simulink library "tqd"  (R2021b)
settings: Solver=VariableStepAuto  StartTime=0.0  StopTime=10.0  RelTol=1e-3
undefined symbols (not defined in the file or in its folder): ATQD_APSDecReq_X_kph, ATQD_APSDecReq_Y_mps2, ATQD_APSDecReqCMD_X_kph, ATQD_APSDecReqTs_X_pct, ATQD_APSDecTimeGain_X_Deg, ATQD_APSDecTimeGain_Y_s, ATQD_APSReqLowSpd_X_Deg, ATQD_AutoHoldReleaseBPS_X_Deg, ATQD_AWDLoadTrqnsGain_X_kg, ATQD_AWDLoadTrqnsGain_Y_pct, ATQD_BOSEnBPSPosn_X_kph, ATQD_BOSMap_X_rpm, ATQD_BOSMap_Y_pct, ATQD_CreepBaseTqD_X_kph, ATQD_CreepBaseTqD_Y_Deg, ATQD_CreepBaseTqR_X_kph, ATQD_CreepBaseTqR_Y_Deg, ATQD_CreepBPSDisPosn_X_Deg, ATQD_CreepBPSDisPosnR_X_Deg, ATQD_CreepBPSEnPosn_X_Deg, ATQD_CreepBPSEnPosnR_X_Deg, ATQD_CreepDeltaTq_X_kph, ATQD_CreepIterm_X_kph, ATQD_CreepIterm_Y_kph, ATQD_CreepItermMaxLimit_X_pct, ATQD_CreepPreloadTime_X_kph, ATQD_CreepPreloadTq_X_kph, ATQD_CreepPreloadTq_Y_s, ATQD_CreepProtTq_X_Deg, ATQD_CreepPterm_X_kph, ATQD_CreepPterm_Y_kph, ATQD_ECOTqMapD_X_rpm, ATQD_ECOTqMapD_Y_pct, ATQD_EOPDTqMapDCon_X_rpm, ATQD_EOPDTqMapDCon_Y_Deg, ATQD_EstInitVehWeight_X_c, ATQD_LHMRollGenMapD_X_rpm, ATQD_LHMRollGenMapD_Y_rpm, ATQD_LHMTqMapD_X_rpm, ATQD_LHMTqMapD_Y_pct, ATQD_NL1TqMapD_X_rpm, ATQD_NL1TqMapD_Y_pct, ATQD_NOPDTqMapDCon_X_rpm, ATQD_NOPDTqMapDCon_Y_Deg, ATQD_NRMRrEDUSpRat_X_rpm, ATQD_NRMRrEDUSpRat_Y_Nm, ATQD_OPDHoldDownRelDelay_X_Deg, ATQD_OPDHoldEnSpd_X_Deg, ATQD_OPDHoldRelDetTime_X_Deg, ATQD_OPDHoldReleaseTq_X_Deg, ATQD_OrigPedTqLowLim_X_Deg, ATQD_OrigPedTqLowLim_Y_pct, ATQD_PedalMapClimbUpLim_X_rpm, ATQD_PedalMapClimbUpLim_Y_Deg, ATQD_PreLoadTq_X_s, ATQD_RollGenMapEL1_X_rpm, ATQD_RollGenMapEL1_Y_rpm, ATQD_SL1TqMapD_X_rpm, ATQD_SL1TqMapD_Y_pct, ATQD_SlideRegenTqGain_X_Gps ... (+491)
libraries: hcu_lib x83, simulink x73, tqr x1
(part 5 of 19)

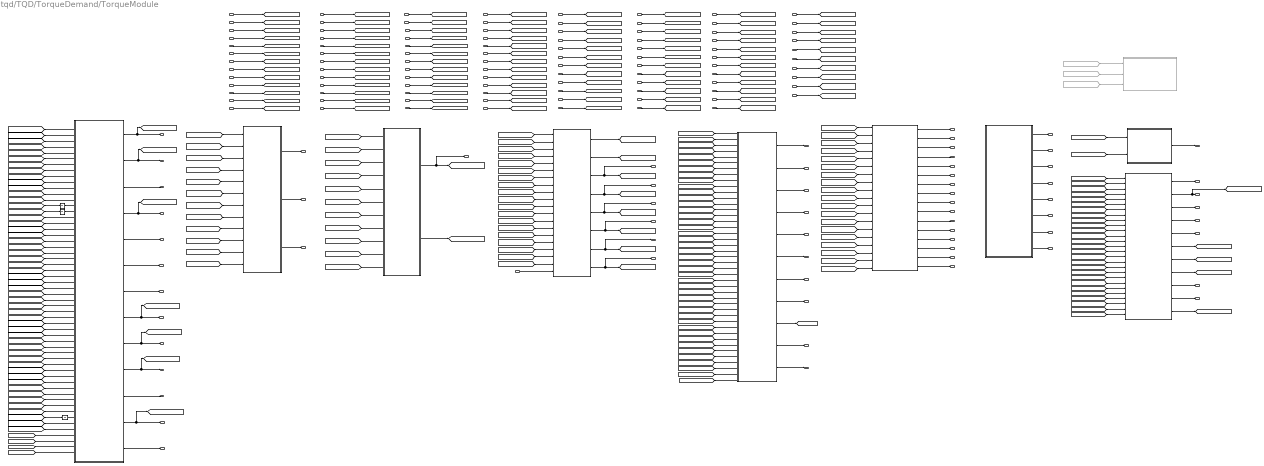
== system tqd/TQD/TorqueDemand/TorqueModule ==
  note: Input Signals
  VTQD_LowIdleAccPedal_flg : Inport
  VPMM_DrivetrainSelect_enum : Inport  Port=2
  VTQD_RollRegenDisableReq_flg : Inport  Port=3
  VTQD_GearActualPosn_enum : Inport  Port=4
  VTQD_CreepON_flg : Inport  Port=5
  VTQD_BrkSwSta_flg : Inport  Port=6
  VTQD_LimpHomeAct_flg : Inport  Port=7
  VTQD_EVDriveMode_enum : Inport  Port=8
  VTQD_RegenMode_enum : Inport  Port=9
  VINP_VehSpeed_kph : Inport  Port=10
  VTQD_TqTargetShaftSpd_rpm : Inport  Port=11
  VTQD_FrShaftSpd_rpm : Inport  Port=12
  VTQD_RrShaftSpd_rpm : Inport  Port=13
  VTQD_ActAPSPosn_pct : Inport  Port=14
  VTQD_ActBPSPosn_pct : Inport  Port=15
  VINP_FrPTCSActive_flg : Inport  Port=16
  VINP_RrPTCSActive_flg : Inport  Port=17
  VINP_FrntAxlTrqReqDrv_Nm : Inport  Port=18
  VINP_RearAxlTrqReqDrv_Nm : Inport  Port=19
  VINP_FrRBCActive_flg : Inport  Port=20
  VINP_RrRBCActive_flg : Inport  Port=21
  VINP_FrntAxlTrqReqBrk_Nm : Inport  Port=22
  VINP_RearAxlTrqReqBrk_Nm : Inport  Port=23
  VVMC_ADASActive_flg : Inport  Port=24
  VVMC_ADASWhlTqReq_Nm : Inport  Port=25
  VVMC_CruzActive_flg : Inport  Port=26
  VVMC_CruzWhlTqReq_Nm : Inport  Port=27
  VVMC_MSAActive_flg : Inport  Port=28
  VVMC_MSAWhlTqReq_Nm : Inport  Port=29
  VVMC_APSActive_flg : Inport  Port=30
  VINP_HVBPwrAvailDchrg_kw : Inport  Port=31
  VTQD_EstVehWeightResult_kg : Inport  Port=32
  VVMC_LongAcc_Gps : Inport  Port=33
  VINP_HVBPwrAvailChrg_kw : Inport  Port=34
  VINP_FrRegenAvailTq_Nm : Inport  Port=35
  VINP_RrRegenAvailTq_Nm : Inport  Port=36
  VINP_FrTMSpd_RPM : Inport  Port=37
  VINP_RrTMSpd_RPM : Inport  Port=38
  VINP_FrEDURealTMTq_Nm : Inport  Port=39
  VINP_RrEDURealTMTq_Nm : Inport  Port=40
  VTQD_ParkRequest_flg : Inport  Port=41
  VPMM_PwrSta_enum : Inport  Port=42
  VTQD_MCUReady4Ext_flg : Inport  Port=43
  VINP_HVBattErr_flg : Inport  Port=44
  VINP_DCDCFaultSta_enum : Inport  Port=45
  VINP_ADASForceIdle_flg : Inport  Port=46
  VTQD_TMRotateDirction_enum : Inport  Port=47
  VINP_LongAccel_Gps : Inport  Port=48
  VTQR_ActualFEDUWhlTqReq_Nm : Inport  Port=49
  VTQR_ActualREDUWhlTqReq_Nm : Inport  Port=50
  VINP_BrkPedalPos_pct : Inport  Port=51
  VTQD_RDCActive_enum : Inport  Port=52
  VVMC_ActMaxSlideRate_pct : Inport  Port=53
  VINP_FrMotorAvailTq_Nm : Inport  Port=54
  VINP_RrMotorAvailTq_Nm : Inport  Port=55
  task_time_s : Inport  Port=56
  VINP_HSAActive_flg : Inport  Port=57
  VTQR_NoABSFEDUWhlTqReq_Nm : Inport  Port=58
  VTQR_NoABSREDUWhlTqReq_Nm : Inport  Port=59
  VINP_AVHActive_flg : Inport  Port=60
  VINP_EPBErrSta_enum : Inport  Port=61
  VVMC_APSSpeedCMD_kph : Inport  Port=62
  VINP_MCUWarnF_enum : Inport  Port=63
  VINP_MCUWarnR_enum : Inport  Port=64
  VVMC_APSReq_enum : Inport  Port=65
  VINP_ACCVehHoldReq_flg : Inport  Port=66
  VTQD_DriveProtRemove_flg : Inport  Port=67
  VINP_ACCRequiredAccel_mps2 : Inport  Port=68
  VVMC_EstSlope_Deg : Inport  Port=69
  VINP_SCPSystemMode_enum : Inport  Port=70
  VINP_SWCResUpSta_flg : Inport  Port=71
  VINP_DrDoorSW_flg : Inport  Port=72
  VINP_PsDoorSW_flg : Inport  Port=73
  VINP_RRDoorSW_flg : Inport  Port=74
  VINP_RLDoorSW_flg : Inport  Port=75
  VINP_HoodSW_flg : Inport  Port=76
  VINP_TailgateSW_flg : Inport  Port=77
  VINP_ADASACCSta_enum : Inport  Port=78
  VINP_EPBSta_enum : Inport  Port=79
  VVMC_ActLRSlideRate_pct : Inport  Port=80
  VVMC_ActRRSlideRate_pct : Inport  Port=81
  VINP_SASAngle_Deg : Inport  Port=82
  VINP_YawRate_degps : Inport  Port=83
  VVMC_ActStESCYaw_degps : Inport  Port=84
  VVMC_CAASActive_flg : Inport  Port=85
  VINP_HVBCellVoltMax_mV : Inport  Port=86
  VINP_HVBCellVoltMin_mV : Inport  Port=87
  VINP_HVBSOH_pct : Inport  Port=88
  VINP_HVBattSOC_pct : Inport  Port=89
  VVMC_RearTqRatio_rat : Inport  Port=90
  VVMC_ACCOvrdMemTq_Nm : Inport  Port=91
  VINP_ESCActive_flg : Inport  Port=92
  VINP_ABSActive_flg : Inport  Port=93
  VINP_IVISnowModeCmd_flg : Inport  Port=94
  VINP_VehicleType_enum : Inport  Port=95
  VDDM_EPB1NoComCFS_flg : Inport  Port=96
  VDDM_EPB1RCErrCFS_flg : Inport  Port=97
  VDDM_EPB1CSErrCFS_flg : Inport  Port=98
  VDDM_EPBSigErrCFS_flg : Inport  Port=99
  ActualWhTqWithDirection : Subsystem  Commented=on
  AvaliableTqLimit : Subsystem
  DriverWhlTqDem : Subsystem
  ExtTqFuncHandShaking : Subsystem
  From45 : From  Commented=on  GotoTag=VTQD_GearActualPosn_enum
  From46 : From  Commented=on  GotoTag=VTQD_AfterAvailableTqDemF_Nm
  From47 : From  Commented=on  GotoTag=VTQD_AfterAvailableTqDemR_Nm
  OPD Hold : Subsystem
  Signal for ESC : Subsystem
  Signals for BCM : Subsystem
  Signals for MCU : Subsystem
  TqCoordination : Subsystem
  TqDistribution : Subsystem
  Unit Delay : UnitDelay  SampleTime=-1  HasFrameUpgradeWarning=on
  Unit Delay1 : UnitDelay  SampleTime=-1  HasFrameUpgradeWarning=on
  Unit Delay2 : UnitDelay  SampleTime=-1  HasFrameUpgradeWarning=on
  VTQD_DriverWhlTqDem_Nm : Outport
  VTQD_TqSourceFr_enum : Outport  Port=2
  VTQD_TqSourceRr_enum : Outport  Port=3
  VTQD_RollRegenEnable_flg : Outport  Port=4
  VTQD_EVDriveModeValid_flg : Outport  Port=5
  VTQD_AfterAvailableTqDemFr_Nm : Outport  Port=6
  VTQD_AfterAvailableTqDemRr_Nm : Outport  Port=7
  VTQD_FrEDUAvailBrkRgnTq_Nm : Outport  Port=8
  VTQD_RrEDUAvailBrkRgnTq_Nm : Outport  Port=9
  VTQD_FrRgnDecrSta_flg : Outport  Port=10
  VTQD_RrRgnDecrSta_flg : Outport  Port=11
  VTQD_FrEDUActTq_Nm : Outport  Port=12
  VTQD_RrEDUActTq_Nm : Outport  Port=13
  VTQD_FrEDURolRgnTq_Nm : Outport  Port=14
  VTQD_RrEDURolRgnTq_Nm : Outport  Port=15
  VTQD_FrEDUSpd_rpm : Outport  Port=16
  VTQD_RrEDUSpd_rpm : Outport  Port=17
  VTQD_FrEDUSpdValid_flg : Outport  Port=18
  VTQD_FrEDUActTqValid_flg : Outport  Port=19
  VTQD_FrEDURolRgnTqValid_flg : Outport  Port=20
  VTQD_FrEDUAvailBrkRgnTqV_flg : Outport  Port=21
  VTQD_RrEDUSpdValid_flg : Outport  Port=22
  VTQD_RrEDUActTqValid_flg : Outport  Port=23
  VTQD_RrEDURolRgnTqValid_flg : Outport  Port=24
  VTQD_RrEDUAvailBrkRgnTqV_flg : Outport  Port=25
  VTQD_RgnAbnorSta_flg : Outport  Port=26
  VTQD_PTCSPermSta_flg : Outport  Port=27
  VTQD_FrRgnPermSta_flg : Outport  Port=28
  VTQD_RrRgnPermSta_flg : Outport  Port=29
  VTQD_DriverWhlTqDemFr_Nm : Outport  Port=30
  VTQD_DriverWhlTqDemRr_Nm : Outport  Port=31
  VTQD_ExternalTqAllow_flg : Outport  Port=32
  VTQD_FrIdcMin_A : Outport  Port=33
  VTQD_FrIdcMax_A : Outport  Port=34
  VTQD_FrUdcMin_V : Outport  Port=35
  VTQD_FrUdcMax_V : Outport  Port=36
  VTQD_RrIdcMin_A : Outport  Port=37
  VTQD_RrIdcMax_A : Outport  Port=38
  VTQD_RrUdcMin_V : Outport  Port=39
  VTQD_RrUdcMax_V : Outport  Port=40
  VTQD_CoordWhlTqDemFr_Nm : Outport  Port=41
  VTQD_CoordWhlTqDemRr_Nm : Outport  Port=42
  VTQD_CreepEnable_flg : Outport  Port=43
  VTQD_ReBrakeLPReq_flg : Outport  Port=44
  VTQD_LoSpdBrkCtrl_flg : Outport  Port=45
  VTQD_BOSEnable_flg : Outport  Port=46
  VTQD_ExtShftAllow_flg : Outport  Port=47
  VTQD_OPDOn2Off_flg : Outport  Port=48
  VTQD_PreLoadHold_flg : Outport  Port=49
  VTQD_PreLoadPreEn_flg : Outport  Port=50
  VTQD_CreepPrLoadEnable_flg : Outport  Port=51
  VTQD_APSStaSys_enum : Outport  Port=52
  VTQD_APSReq_enum : Outport  Port=53
  VTQD_APSDecReqA_flg : Outport  Port=54
  VTQD_APSDecReq_mps2 : Outport  Port=55
  VTQD_ActParkRequest_flg : Outport  Port=56
  VTQD_RegenTqLimitEn_flg : Outport  Port=57
  VTQD_ExtDoorAllow_flg : Outport  Port=58
  VTQD_WhlTqCapGenFr_Nm : Outport  Port=59
  VTQD_WhlTqCapGenRr_Nm : Outport  Port=60
  VTQD_OPDHoldAllowPark_flg : Outport  Port=61
  VTQD_OPDHoldLamp_flg : Outport  Port=62
  VTQD_CreepBaseTqD_Nm : Outport  Port=63
  VTQD_VehActSpd_kph : Outport  Port=64
  VTQD_CoordTqDem_Nm : Outport  Port=65
  wires:
  VTQD_ActAPSPosn_pct/1 -> [VTQD_ActAPSPosn_pct]
  VTQD_GearActualPosn_enum/1 -> [VTQD_GearActualPosn_enum]
  VINP_VehSpeed_kph/1 -> [VINP_VehSpeed_kph]
  VTQD_BrkSwSta_flg/1 -> [VTQD_BrkSwSta_flg]
  VTQD_RegenMode_enum/1 -> [VTQD_RegenMode_enum]
  VINP_FrntAxlTrqReqDrv_Nm/1 -> [VINP_FrntAxlTrqReqDrv_Nm]
  VINP_RearAxlTrqReqDrv_Nm/1 -> [VINP_RearAxlTrqReqDrv_Nm]
  VINP_FrPTCSActive_flg/1 -> [VINP_FrPTCSActive_flg]
  VINP_FrntAxlTrqReqBrk_Nm/1 -> [VINP_FrntAxlTrqReqBrk_Nm]
  VINP_RearAxlTrqReqBrk_Nm/1 -> [VINP_RearAxlTrqReqBrk_Nm]
  VTQD_RollRegenDisableReq_flg/1 -> [VTQD_RollRegenDisableReq_flg]
  VINP_FrRBCActive_flg/1 -> [VINP_FrRBCActive_flg]
  VTQD_ActBPSPosn_pct/1 -> [VTQD_ActBPSPosn_pct]
  VVMC_CruzWhlTqReq_Nm/1 -> [VVMC_CruzWhlTqReq_Nm]
  VVMC_CruzActive_flg/1 -> [VVMC_CruzActive_flg]
  VTQD_EVDriveMode_enum/1 -> [VTQD_EVDriveMode_enum]
  VTQD_LimpHomeAct_flg/1 -> [VTQD_LimpHomeAct_flg]
  VTQD_CreepON_flg/1 -> [VTQD_CreepON_flg]
  VTQD_TqTargetShaftSpd_rpm/1 -> [VTQD_TqTargetShaftSpd_rpm]
  VPMM_DrivetrainSelect_enum/1 -> [VPMM_DrivetrainSelect_enum]
  [VTQD_TqTargetShaftSpd_rpm] -> DriverWhlTqDem/10(VTQD_TqTargetShaftSpd_rpm)
  [VTQD_LimpHomeAct_flg] -> DriverWhlTqDem/6(VTQD_LimpHomeAct_flg)
  [VTQD_EVDriveMode_enum] -> DriverWhlTqDem/7(VTQD_EVDriveMode_enum)
  [VTQD_RegenMode_enum] -> DriverWhlTqDem/8(VTQD_RegenMode_enum)
  [VTQD_CreepON_flg] -> DriverWhlTqDem/4("VTQD_CreepON_flg ")
  [VTQD_GearActualPosn_enum] -> DriverWhlTqDem/3(VTQD_GearActualPosn_enum)
  [VTQD_LowIdleAccPedal_flg] -> DriverWhlTqDem/1(VDHP_LowIdleAccPedal_flg)
  [VTQD_ActAPSPosn_pct] -> DriverWhlTqDem/11(VTQD_ActAPSPosn_pct)
  TqDistribution/2(VTQD_RrEDUSpRat_rat) -> [VTQD_RrEDUSpRat_rat]
  TqDistribution/1(VTQD_FrEDUSpRat_rat) -> [VTQD_FrEDUSpRat_rat]
  VINP_HVBPwrAvailChrg_kw/1 -> [VINP_HVBPwrAvailChrg_kw]
  VINP_HVBPwrAvailDchrg_kw/1 -> [VINP_HVBPwrAvailDchrg_kw]
  DriverWhlTqDem/1(VTQD_DriverWhlTqDem_Nm) -> VTQD_DriverWhlTqDem_Nm/1, [VTQD_DriverWhlTqDem_Nm]
  [VPMM_DrivetrainSelect_enum] -> TqDistribution/1(VPMM_DrivetrainSelect_enum)
  VVMC_MSAActive_flg/1 -> [VVMC_MSAActive_flg]
  VVMC_MSAWhlTqReq_Nm/1 -> [VVMC_MSAWhlTqReq_Nm]
  VVMC_APSActive_flg/1 -> [VVMC_APSActive_flg]
  VVMC_ADASActive_flg/1 -> [VVMC_ADASActive_flg]
  VVMC_ADASWhlTqReq_Nm/1 -> [VVMC_ADASWhlTqReq_Nm]
  [VTQD_BrkSwSta_flg] -> DriverWhlTqDem/5(VTQD_BrkSwSta_flg)
  [VTQD_ActBPSPosn_pct] -> DriverWhlTqDem/12(VTQD_ActBPSPosn_pct)
  [VINP_VehSpeed_kph] -> DriverWhlTqDem/9(VINP_VehSpeed_kph)
  [VTQD_RollRegenDisableReq_flg] -> DriverWhlTqDem/2(VTQD_RollRegenDisableReq_flg)
  From46/1 -> ActualWhTqWithDirection/2(VTQD_AfterAvailableTqDemF_Nm)
  From45/1 -> ActualWhTqWithDirection/1(VTQD_GearActualPosn_enum)
  From47/1 -> ActualWhTqWithDirection/3(VTQD_AfterAvailableTqDemR_Nm)
  VTQD_FrShaftSpd_rpm/1 -> [VTQD_FrShaftSpd_rpm]
  VTQD_RrShaftSpd_rpm/1 -> [VTQD_RrShaftSpd_rpm]
  VTQD_LowIdleAccPedal_flg/1 -> [VTQD_LowIdleAccPedal_flg]
  DriverWhlTqDem/2(VTQD_RollRegenEnable_flg) -> VTQD_RollRegenEnable_flg/1, [VTQD_RollRegenEnable_flg]
  DriverWhlTqDem/3(VTQD_EVDriveModeValid_flg) -> VTQD_EVDriveModeValid_flg/1
  VINP_RrPTCSActive_flg/1 -> [VINP_RrPTCSActive_flg]
  VINP_RrRBCActive_flg/1 -> [VINP_RrRBCActive_flg]
  VINP_RrTMSpd_RPM/1 -> [VINP_RrTMSpd_rpm]
  VINP_FrTMSpd_RPM/1 -> [VINP_FrTMSpd_rpm]
  VINP_RrRegenAvailTq_Nm/1 -> [VINP_RrRegenAvailTq_Nm]
  VINP_FrRegenAvailTq_Nm/1 -> [VINP_FrRegenAvailTq_Nm]
  VINP_RrEDURealTMTq_Nm/1 -> [VINP_RrEDURealTMTq_Nm]
  VINP_FrEDURealTMTq_Nm/1 -> [VINP_FrEDURealTMTq_Nm]
  AvaliableTqLimit/8(VTQD_RrRgnPermSta_flg) -> VTQD_RrRgnPermSta_flg/1  "VTQD_RrRgnPermSta_flg"
  AvaliableTqLimit/6(VTQD_RrRgnDecrSta_flg) -> VTQD_RrRgnDecrSta_flg/1  "VTQD_RrRgnDecrSta_flg"
  Signal for ESC/4(VTQD_RrEDURolRgnTq_Nm) -> VTQD_RrEDURolRgnTq_Nm/1
  AvaliableTqLimit/7(VTQD_FrRgnPermSta_flg) -> VTQD_FrRgnPermSta_flg/1  "VTQD_FrRgnPermSta_flg"
  [VTQD_RrShaftSpd_rpm] -> AvaliableTqLimit/2(VTQD_RrShaftSpd_rpm)
  Signal for ESC/2(VTQD_RrEDUActTq_Nm) -> VTQD_RrEDUActTq_Nm/1
  Signal for ESC/9(VTQD_FrEDURolRgnTqValid_flg) -> VTQD_FrEDURolRgnTqValid_flg/1  "VTQD_FrEDURolRgnTqValid_flg"
  Signal for ESC/16(VTQD_PTCSPermSta_flg) -> VTQD_PTCSPermSta_flg/1
  Signal for ESC/6(VTQD_RrEDUSpd_rpm) -> VTQD_RrEDUSpd_rpm/1
  Signal for ESC/1(VTQD_FrEDUActTq_Nm) -> VTQD_FrEDUActTq_Nm/1
  [VINP_RrRegenAvailTq_Nm] -> AvaliableTqLimit/14(VINP_RrRegenAvailTq_Nm)
  Signal for ESC/13(VTQD_RrEDURolRgnTqValid_flg) -> VTQD_RrEDURolRgnTqValid_flg/1  "VTQD_RrEDURolRgnTqValid_flg"
  [VINP_HVBPwrAvailChrg_kw] -> AvaliableTqLimit/4(VINP_HVBPwrAvailChrg_kw)
  [VTQD_FrShaftSpd_rpm] -> AvaliableTqLimit/1(VTQD_FrShaftSpd_rpm)
  AvaliableTqLimit/1(VTQD_AfterAvailableTqDemFr_Nm) -> VTQD_AfterAvailableTqDemFr_Nm/1
  Signal for ESC/8(VTQD_FrEDUActTqValid_flg) -> VTQD_FrEDUActTqValid_flg/1  "VTQD_FrEDUActTqValid_flg"
  Signal for ESC/12(VTQD_RrEDUActTqValid_flg) -> VTQD_RrEDUActTqValid_flg/1  "VTQD_RrEDUActTqValid_flg"
  [VINP_HVBPwrAvailDchrg_kw] -> AvaliableTqLimit/3(VINP_HVBPwrAvailDchrg_kw)
  Signal for ESC/15(VTQD_RgnAbnorSta_flg) -> VTQD_RgnAbnorSta_flg/1
  Signal for ESC/11(VTQD_RrEDUSpdValid_flg) -> VTQD_RrEDUSpdValid_flg/1  "VTQD_RrEDUSpdValid_flg"
  Signal for ESC/3(VTQD_FrEDURolRgnTq_Nm) -> VTQD_FrEDURolRgnTq_Nm/1
  [VINP_FrRegenAvailTq_Nm] -> AvaliableTqLimit/13(VINP_FrRegenAvailTq_Nm)
  AvaliableTqLimit/5(VTQD_FrRgnDecrSta_flg) -> VTQD_FrRgnDecrSta_flg/1  "VTQD_FrRgnDecrSta_flg"
  AvaliableTqLimit/2(VTQD_AfterAvailableTqDemRr_Nm) -> VTQD_AfterAvailableTqDemRr_Nm/1
  AvaliableTqLimit/3(VTQD_FrEDUAvailBrkRgnTq_Nm) -> VTQD_FrEDUAvailBrkRgnTq_Nm/1
  [VTQD_CoordWhlTqDemRr_Nm] -> AvaliableTqLimit/6(VTQD_CoordWhlTqDemRr_Nm)
  Signal for ESC/14(VTQD_RrEDUAvailBrkRgnTqV_flg) -> VTQD_RrEDUAvailBrkRgnTqV_flg/1  "VTQD_RrEDUAvailBrkRgnTqV_flg"
  [VTQD_DriverWhlTqDemFr_Nm] -> AvaliableTqLimit/11(VTQD_DriverWhlTqDemFr_Nm)
  [VTQD_CoordWhlTqDemFr_Nm] -> AvaliableTqLimit/5(VTQD_CoordWhlTqDemFr_Nm)
  [VTQD_DriverWhlTqDemRr_Nm] -> AvaliableTqLimit/12(VTQD_DriverWhlTqDemRr_Nm)
  [VTQD_FrEDUSpRat_rat] -> AvaliableTqLimit/7(VTQD_FrEDUSpRat_rat)
  [VTQD_RrEDUSpRat_rat] -> AvaliableTqLimit/8(VTQD_RrEDUSpRat_rat)
  Signal for ESC/5(VTQD_FrEDUSpd_rpm) -> VTQD_FrEDUSpd_rpm/1
  AvaliableTqLimit/4(VTQD_RrEDUAvailBrkRgnTq_Nm) -> VTQD_RrEDUAvailBrkRgnTq_Nm/1
  [VTQD_TqSourceRr_enum] -> AvaliableTqLimit/10(VTQD_TqSourceRr_enum)
  [VTQD_TqSourceFr_enum] -> AvaliableTqLimit/9(VTQD_TqSourceFr_enum)
  Signal for ESC/7(VTQD_FrEDUSpdValid_flg) -> VTQD_FrEDUSpdValid_flg/1  "VTQD_FrEDUSpdValid_flg"
  [VINP_DCDCFaultSta_enum] -> ExtTqFuncHandShaking/4(VINP_DCDCFaultSta_enum)
  [VINP_HVBattErr_flg] -> ExtTqFuncHandShaking/3(VINP_HVBattErr_flg)
  [VTQD_MCUReady4Ext_flg] -> ExtTqFuncHandShaking/2(VTQD_MCUReady4Ext_flg)
  [VPMM_PwrSta_enum] -> ExtTqFuncHandShaking/1(VPMM_PwrSta_enum)
  VINP_HVBattErr_flg/1 -> [VINP_HVBattErr_flg]
  VINP_ADASForceIdle_flg/1 -> [VINP_ADASForceIdle_flg]
  VTQD_MCUReady4Ext_flg/1 -> [VTQD_MCUReady4Ext_flg]
  VPMM_PwrSta_enum/1 -> [VPMM_PwrSta_enum]
  VINP_DCDCFaultSta_enum/1 -> [VINP_DCDCFaultSta_enum]
  ExtTqFuncHandShaking/1(VTQD_ExternalTqAllow_flg) -> VTQD_ExternalTqAllow_flg/1
  VTQD_TMRotateDirction_enum/1 -> [VTQD_TMRotateDirction_enum]
  [VTQD_TMRotateDirction_enum] -> DriverWhlTqDem/13(VTQD_TMRotateDirction_enum)
  Signals for MCU/8(VTQD_RrUdcMax_V) -> VTQD_RrUdcMax_V/1
  Signals for MCU/5(VTQD_RrIdcMin_A) -> VTQD_RrIdcMin_A/1
  Signals for MCU/3(VTQD_FrUdcMin_V) -> VTQD_FrUdcMin_V/1
  Signals for MCU/2(VTQD_FrIdcMax_A) -> VTQD_FrIdcMax_A/1
  Signals for MCU/7(VTQD_RrUdcMin_V) -> VTQD_RrUdcMin_V/1
  Signals for MCU/6(VTQD_RrIdcMax_A) -> VTQD_RrIdcMax_A/1
  Signals for MCU/4(VTQD_FrUdcMax_V) -> VTQD_FrUdcMax_V/1
  Signals for MCU/1(VTQD_FrIdcMin_A) -> VTQD_FrIdcMin_A/1
  [VTQD_TqSourceFr_enum] -> Unit Delay/1
  [VTQD_TqSourceRr_enum] -> Unit Delay1/1
  Unit Delay/1 -> DriverWhlTqDem/14(VTQD_TqSourceFr_enum)
  Unit Delay1/1 -> DriverWhlTqDem/15(VTQD_TqSourceRr_enum)
  DriverWhlTqDem/4(VTQD_CreepEnable_flg) -> [VTQD_CreepEnable_flg], VTQD_CreepEnable_flg/1
  [VTQD_DriverWhlTqDem_Nm] -> AvaliableTqLimit/15(VTQD_DriverWhlTqDem_Nm)
  VINP_LongAccel_Gps/1 -> [VINP_LongAccel_Gps]
  [VINP_LongAccel_Gps] -> Signals for BCM/2(VINP_LongAccel_Gps)
  Signals for BCM/1(VTQD_ReBrakeLPReq_flg) -> VTQD_ReBrakeLPReq_flg/1
  AvaliableTqLimit/9(VTQD_ARegenActive_flg) -> [VTQD_ARegenActive_flg]
  [VTQD_ARegenActive_flg] -> Signals for BCM/1(VTQD_ARegenActive_flg)
  VTQR_ActualFEDUWhlTqReq_Nm/1 -> [VTQR_ActualFEDUWhlTqReq_Nm]
  VTQR_ActualREDUWhlTqReq_Nm/1 -> [VTQR_ActualREDUWhlTqReq_Nm]
  VINP_BrkPedalPos_pct/1 -> [VINP_BrkPedalPos_pct]
  VTQD_RDCActive_enum/1 -> [VTQD_RDCActive_enum]
  [VTQD_RDCActive_enum] -> DriverWhlTqDem/17(VTQD_RDCActive_enum)
  VVMC_ActMaxSlideRate_pct/1 -> [VVMC_ActMaxSlideRate_pct]
  VINP_RrMotorAvailTq_Nm/1 -> [VINP_RrMotorAvailTq_Nm]
  VINP_FrMotorAvailTq_Nm/1 -> [VINP_FrMotorAvailTq_Nm]
  [VINP_FrMotorAvailTq_Nm] -> AvaliableTqLimit/16(VINP_FrMotorAvailTq_Nm)
  [VINP_RrMotorAvailTq_Nm] -> AvaliableTqLimit/17(VINP_RrMotorAvailTq_Nm)
  [VTQD_CreepEnable_flg] -> AvaliableTqLimit/18(VTQD_CreepEnable_flg)
  [VINP_FrEDURealTMTq_Nm] -> Signal for ESC/1(VINP_FrEDURealTMTq_Nm)
  [VINP_RrEDURealTMTq_Nm] -> Signal for ESC/2(VINP_RrEDURealTMTq_Nm)
  [VTQD_RollRegenEnable_flg] -> Signal for ESC/3(VTQD_RollRegenEnable_flg)
  [VINP_MCUWarnR_enum] -> Signal for ESC/9(VINP_MCUWarnR_enum)
  [VINP_MCUWarnF_enum] -> Signal for ESC/8(VINP_MCUWarnF_enum)
  [VVMC_ADASActive_flg] -> TqCoordination/2(VVMC_ADASActive_flg)
  [VINP_ADASForceIdle_flg] -> TqCoordination/10(VINP_ADASForceIdle_flg)
  [VTQD_GearActualPosn_enum] -> TqCoordination/1(VTQD_GearActualPosn_enum)
  [VVMC_MSAWhlTqReq_Nm] -> TqCoordination/7(VVMC_MSAWhlTqReq_Nm)
  [VTQD_DriverWhlTqDem_Nm] -> TqCoordination/9(VTQD_DriverWhlTqDem_Nm)
  [VVMC_CruzActive_flg] -> TqCoordination/4(VVMC_CruzActive_flg)
  [VVMC_APSActive_flg] -> TqCoordination/8(VVMC_APSActive_flg)
  [VVMC_ADASWhlTqReq_Nm] -> TqCoordination/3(VVMC_ADASWhlTqReq_Nm)
  [VVMC_CruzWhlTqReq_Nm] -> TqCoordination/5(VVMC_CruzWhlTqReq_Nm)
  [VVMC_MSAActive_flg] -> TqCoordination/6(VVMC_MSAActive_flg)
  task_time_s/1 -> [task_time_s]
  [task_time_s] -> DriverWhlTqDem/18(task_time_s)
  DriverWhlTqDem/5(VTQD_LoSpdBrkCtrl_flg) -> VTQD_LoSpdBrkCtrl_flg/1
  Signal for ESC/10(VTQD_FrEDUAvailBrkRgnTqV_flg) -> VTQD_FrEDUAvailBrkRgnTqV_flg/1  "VTQD_FrEDUAvailBrkRgnTqV_flg"
  DriverWhlTqDem/6(VTQD_BOSEnable_flg) -> VTQD_BOSEnable_flg/1
  VINP_HSAActive_flg/1 -> [VINP_HSAActive_flg]
  VTQR_NoABSFEDUWhlTqReq_Nm/1 -> [VTQR_NoABSFEDUWhlTqReq_Nm]
  VTQR_NoABSREDUWhlTqReq_Nm/1 -> [VTQR_NoABSREDUWhlTqReq_Nm]
  VINP_AVHActive_flg/1 -> [VINP_AVHActive_flg]
  VINP_MCUWarnF_enum/1 -> [VINP_MCUWarnF_enum]
  VINP_MCUWarnR_enum/1 -> [VINP_MCUWarnR_enum]
  VINP_EPBErrSta_enum/1 -> [VINP_EPBErrSta_enum]
  VVMC_APSSpeedCMD_kph/1 -> [VVMC_APSSpeedCMD_kph]
  [VINP_HSAActive_flg] -> DriverWhlTqDem/19(VINP_HSAActive_flg)
  [VINP_RrRBCActive_flg] -> DriverWhlTqDem/20(VINP_RrRBCActive_flg)
  [VINP_FrRBCActive_flg] -> DriverWhlTqDem/21(VINP_FrRBCActive_flg)
  [VVMC_ADASActive_flg] -> DriverWhlTqDem/22(VVMC_ADASActive_flg)
  [VTQD_APSReq_enum] -> DriverWhlTqDem/23(VTQD_APSReq_enum)
  [VINP_AVHActive_flg] -> DriverWhlTqDem/24(VINP_AVHActive_flg)
  [VVMC_APSSpeedCMD_kph] -> DriverWhlTqDem/25(VVMC_APSSpeedCMD_kph)
  [VVMC_APSActive_flg] -> DriverWhlTqDem/26(VVMC_APSActive_flg)
  [VINP_EPBErrSta_enum] -> ExtTqFuncHandShaking/5(VINP_EPBErrSta_enum)
  ExtTqFuncHandShaking/2(VTQD_ExtShftAllow_flg) -> VTQD_ExtShftAllow_flg/1
  [VINP_FrntAxlTrqReqBrk_Nm] -> Signal for ESC/4(VINP_FrntAxlTrqReqBrk_Nm)
  [VINP_RearAxlTrqReqBrk_Nm] -> Signal for ESC/5(VINP_RearAxlTrqReqBrk_Nm)
  [VINP_FrRBCActive_flg] -> Signal for ESC/10(VINP_FrRBCActive_flg)
  [VINP_RrRBCActive_flg] -> Signal for ESC/11(VINP_RrRBCActive_flg)
  [VTQR_ActualFEDUWhlTqReq_Nm] -> Signal for ESC/12(VTQR_ActualFEDUWhlTqReq_Nm)
  [VTQR_ActualREDUWhlTqReq_Nm] -> Signal for ESC/13(VTQR_ActualREDUWhlTqReq_Nm)
  [VTQR_NoABSFEDUWhlTqReq_Nm] -> Signal for ESC/14(VTQR_NoABSFEDUWhlTqReq_Nm)
  [VTQR_NoABSREDUWhlTqReq_Nm] -> Signal for ESC/15(VTQR_NoABSREDUWhlTqReq_Nm)
  [VTQD_DriverWhlTqDem_Nm] -> Signal for ESC/16(VTQD_DriverWhlTqDem_Nm)
  [VINP_FrTMSpd_rpm] -> Signal for ESC/6(VINP_FrTMSpd_rpm)
  [VINP_RrTMSpd_rpm] -> Signal for ESC/7(VINP_RrTMSpd_rpm)
  DriverWhlTqDem/7(VTQD_OPDOn2Off_flg) -> VTQD_OPDOn2Off_flg/1
  [VINP_FrEDURealTMTq_Nm] -> DriverWhlTqDem/27(VINP_FrEDURealTMTq_Nm)
  [VINP_RrEDURealTMTq_Nm] -> DriverWhlTqDem/28(VINP_RrEDURealTMTq_Nm)
  DriverWhlTqDem/9(VTQD_PreLoadPreEn_flg) -> [VTQD_PreLoadPreEn_flg], VTQD_PreLoadPreEn_flg/1
  [VVMC_ADASActive_flg] -> AvaliableTqLimit/19(VVMC_ADASActive_flg)
  DriverWhlTqDem/10(VTQD_CreepPrLoadEnable_flg) -> [VTQD_CreepPrLoadEnable_flg], VTQD_CreepPrLoadEnable_flg/1
  [VVMC_ADASActive_flg] -> Signal for ESC/17(VVMC_ADASActive_flg)
  VINP_ACCVehHoldReq_flg/1 -> [VINP_ACCVehHoldReq_flg]
  VVMC_APSReq_enum/1 -> [VVMC_APSReq_enum]
  DriverWhlTqDem/8(VTQD_PreLoadHold_flg) -> [VTQD_PreLoadHold_flg], VTQD_PreLoadHold_flg/1
  [VTQD_PreLoadHold_flg] -> TqCoordination/11(VTQD_PreLoadHold_flg)
  VTQD_DriveProtRemove_flg/1 -> [VTQD_DriveProtRemove_flg]
  VINP_ACCRequiredAccel_mps2/1 -> [VINP_ACCRequiredAccel_mps2]
  [VINP_ACCRequiredAccel_mps2] -> Signal for ESC/18(VINP_ACCRequiredAccel_mps2)
  VTQD_EstVehWeightResult_kg/1 -> [VTQD_EstVehWeightResult_kg]
  VVMC_LongAcc_Gps/1 -> [VVMC_LongAcc_Gps]
  VTQD_ParkRequest_flg/1 -> [VTQD_ParkRequest_flg]
  [VINP_ACCVehHoldReq_flg] -> DriverWhlTqDem/29(VINP_ACCVehHoldReq_flg)
  [VVMC_APSReq_enum] -> DriverWhlTqDem/30(VVMC_APSReq_enum)
  [VTQD_RrShaftSpd_rpm] -> TqDistribution/2(VTQD_RrShaftSpd_rpm)
  [VTQD_DriverWhlTqDem_Nm] -> TqDistribution/3(VTQD_DriverWhlTqDem_Nm)
  [VTQD_EVDriveMode_enum] -> TqDistribution/4(VTQD_EVDriveMode_enum)
  [VTQD_LimpHomeAct_flg] -> TqDistribution/5(VTQD_LimpHomeAct_flg)
  [VVMC_APSActive_flg] -> TqDistribution/6(VVMC_APSActive_flg)
  [VTQD_CreepPrLoadEnable_flg] -> TqDistribution/7(VTQD_CreepPrLoadEnable_flg)
  [VTQD_EstVehWeightResult_kg] -> TqDistribution/8(VTQD_EstVehWeightResult_kg)
  [VTQD_ActBPSPosn_pct] -> OPD Hold/5(VTQD_ActBPSPosn_pct)
  OPD Hold/3(VTQD_APSDecReqA_flg) -> VTQD_APSDecReqA_flg/1
  OPD Hold/5(VTQD_ActParkRequest_flg) -> VTQD_ActParkRequest_flg/1
  OPD Hold/4(VTQD_APSDecReq_mps2) -> VTQD_APSDecReq_mps2/1
  [VVMC_CruzActive_flg] -> OPD Hold/7(VVMC_CruzActive_flg)
  [VTQD_ParkRequest_flg] -> OPD Hold/8(VTQD_ParkRequest_flg)
  [VVMC_ADASActive_flg] -> OPD Hold/6(VVMC_ADASActive_flg)
  [VTQD_RegenMode_enum] -> OPD Hold/2(VTQD_RegenMode_enum)
  OPD Hold/1(VTQD_APSStaSys_enum) -> VTQD_APSStaSys_enum/1
  [task_time_s] -> OPD Hold/1(task_time_s)
  OPD Hold/2(VTQD_APSReq_enum) -> [VTQD_APSReq_enum], VTQD_APSReq_enum/1
  [VTQD_GearActualPosn_enum] -> OPD Hold/3(VTQD_GearActualPosn_enum)
  [VTQD_DriveProtRemove_flg] -> AvaliableTqLimit/20(VTQD_DriveProtRemove_flg)
  [VINP_RearAxlTrqReqDrv_Nm] -> AvaliableTqLimit/24(VINP_RearAxlTrqReqDrv_Nm)
  [VINP_FrntAxlTrqReqDrv_Nm] -> AvaliableTqLimit/23(VINP_FrntAxlTrqReqDrv_Nm)
  [VINP_RrPTCSActive_flg] -> AvaliableTqLimit/22(VINP_RrPTCSActive_flg)
  [VINP_FrPTCSActive_flg] -> AvaliableTqLimit/21(VINP_FrPTCSActive_flg)
  [VVMC_ActMaxSlideRate_pct] -> DriverWhlTqDem/16(VVMC_ActMaxSlideRate_pct)
  VVMC_EstSlope_Deg/1 -> [VVMC_EstSlope_Deg]
  [VVMC_LongAcc_Gps] -> DriverWhlTqDem/31(VVMC_LongAcc_Gps)
  DriverWhlTqDem/11(VTQD_RegenTqLimitEn_flg) -> VTQD_RegenTqLimitEn_flg/1
  [VVMC_EstSlope_Deg] -> OPD Hold/9(VVMC_EstSlope_Deg)
  [VVMC_EstSlope_Deg] -> DriverWhlTqDem/32(VVMC_EstSlope_Deg)
  [VINP_SCPSystemMode_enum] -> DriverWhlTqDem/33(VINP_SCPSystemMode_enum)
  [VPMM_PwrSta_enum] -> DriverWhlTqDem/34(VPMM_PwrSta_enum)
  [VINP_SWCResUpSta_flg] -> DriverWhlTqDem/35(VINP_SWCResUpSta_flg)
  [VINP_BrkPedalPos_pct] -> DriverWhlTqDem/36(VINP_BrkPedalPos_pct)
  [VTQR_NoABSFEDUWhlTqReq_Nm] -> DriverWhlTqDem/37(VTQR_NoABSFEDUWhlTqReq_Nm)
  [VTQR_NoABSREDUWhlTqReq_Nm] -> DriverWhlTqDem/38(VTQR_NoABSREDUWhlTqReq_Nm)
  [VTQD_APSReqTimer_s] -> DriverWhlTqDem/39(VTQD_APSReqTimer_s)
  [VINP_FrPTCSActive_flg] -> DriverWhlTqDem/40(VINP_FrPTCSActive_flg)
  [VINP_RrPTCSActive_flg] -> DriverWhlTqDem/41(VINP_RrPTCSActive_flg)
  [VINP_ADASACCSta_enum] -> DriverWhlTqDem/42(VINP_ADASACCSta_enum)
  [VINP_EPBSta_enum] -> DriverWhlTqDem/43(VINP_EPBSta_enum)
  DriverWhlTqDem/12(VTQD_VehActSpd_kph) -> [VTQD_VehActSpd_kph], VTQD_VehActSpd_kph/1
  [VINP_DrDoorSW_flg] -> ExtTqFuncHandShaking/6(VINP_DrDoorSW_flg)
  [VINP_PsDoorSW_flg] -> ExtTqFuncHandShaking/7(VINP_PsDoorSW_flg)
  [VINP_RRDoorSW_flg] -> ExtTqFuncHandShaking/8(VINP_RRDoorSW_flg)
  [VINP_RLDoorSW_flg] -> ExtTqFuncHandShaking/9(VINP_RLDoorSW_flg)
  [VINP_HoodSW_flg] -> ExtTqFuncHandShaking/10(VINP_HoodSW_flg)
  [VINP_TailgateSW_flg] -> ExtTqFuncHandShaking/11(VINP_TailgateSW_flg)
  ExtTqFuncHandShaking/3(VTQD_ExtDoorAllow_flg) -> VTQD_ExtDoorAllow_flg/1
  TqCoordination/1(VTQD_CoordTqDem_Nm) -> VTQD_CoordTqDem_Nm/1, [VTQD_CoordTqDem_Nm]
  TqCoordination/2(VTQD_TqSource_enum) -> [VTQD_TqSource_enum]
  [VTQD_CoordTqDem_Nm] -> TqDistribution/9(VTQD_CoordTqDem_Nm)
  [VTQD_TqSource_enum] -> TqDistribution/10(VTQD_TqSource_enum)
  [VINP_FrRBCActive_flg] -> TqDistribution/11(VINP_FrRBCActive_flg)
  [VINP_RrRBCActive_flg] -> TqDistribution/12(VINP_RrRBCActive_flg)
  [VTQD_RollRegenEnable_flg] -> TqDistribution/13(VTQD_RollRegenEnable_flg)
  [VINP_FrPTCSActive_flg] -> TqDistribution/14(VINP_FrPTCSActive_flg)
  [VINP_RrPTCSActive_flg] -> TqDistribution/15(VINP_RrPTCSActive_flg)
  [VINP_FrntAxlTrqReqDrv_Nm] -> TqDistribution/16(VINP_FrntAxlTrqReqDrv_Nm)
  [VINP_RearAxlTrqReqDrv_Nm] -> TqDistribution/17(VINP_RearAxlTrqReqDrv_Nm)
  TqDistribution/3(VTQD_CoordWhlTqDemFr_Nm) -> VTQD_CoordWhlTqDemFr_Nm/1, [VTQD_CoordWhlTqDemFr_Nm]
  TqDistribution/4(VTQD_CoordWhlTqDemRr_Nm) -> VTQD_CoordWhlTqDemRr_Nm/1, [VTQD_CoordWhlTqDemRr_Nm]
  TqDistribution/5(VTQD_TqSourceFr_enum) -> VTQD_TqSourceFr_enum/1, [VTQD_TqSourceFr_enum]
  TqDistribution/6(VTQD_TqSourceRr_enum) -> VTQD_TqSourceRr_enum/1, [VTQD_TqSourceRr_enum]
  TqDistribution/7(VTQD_DriverWhlTqDemFr_Nm) -> VTQD_DriverWhlTqDemFr_Nm/1, [VTQD_DriverWhlTqDemFr_Nm]
  TqDistribution/8(VTQD_DriverWhlTqDemRr_Nm) -> VTQD_DriverWhlTqDemRr_Nm/1, [VTQD_DriverWhlTqDemRr_Nm]
  [VTQD_VehActSpd_kph] -> OPD Hold/4(VTQD_VehActSpd_kph)
  [VVMC_LongAcc_Gps] -> OPD Hold/10(VVMC_LongAcc_Gps)
  OPD Hold/6(VTQD_APSReqTimer_s) -> [VTQD_APSReqTimer_s]
  VINP_SWCResUpSta_flg/1 -> [VINP_SWCResUpSta_flg]
  VINP_SCPSystemMode_enum/1 -> [VINP_SCPSystemMode_enum]
  VINP_RLDoorSW_flg/1 -> [VINP_RLDoorSW_flg]
  VINP_HoodSW_flg/1 -> [VINP_HoodSW_flg]
  VINP_TailgateSW_flg/1 -> [VINP_TailgateSW_flg]
  VINP_DrDoorSW_flg/1 -> [VINP_DrDoorSW_flg]
  VINP_PsDoorSW_flg/1 -> [VINP_PsDoorSW_flg]
  VINP_RRDoorSW_flg/1 -> [VINP_RRDoorSW_flg]
  VINP_ADASACCSta_enum/1 -> [VINP_ADASACCSta_enum]
  VINP_EPBSta_enum/1 -> [VINP_EPBSta_enum]
  OPD Hold/7(VTQD_OPDHoldEnRel_flg) -> [VTQD_OPDHoldEnRel_flg]
  [VTQD_OPDHoldEnRel_flg] -> DriverWhlTqDem/44(VTQD_OPDHoldEnRel_flg)
  [VTQD_GearActualPosn_enum] -> AvaliableTqLimit/25(VTQD_GearActualPosn_enum)
  [VTQD_LowIdleAccPedal_flg] -> AvaliableTqLimit/27(VTQD_LowIdleAccPedal_flg)
  [VTQD_VehActSpd_kph] -> AvaliableTqLimit/28(VTQD_VehActSpd_kph)
  [VINP_RrTMSpd_rpm] -> AvaliableTqLimit/29(VINP_RrTMSpd_rpm)
  [VINP_FrTMSpd_rpm] -> AvaliableTqLimit/30(VINP_FrTMSpd_rpm)
  [task_time_s] -> AvaliableTqLimit/31(task_time_s)
  [VPMM_DrivetrainSelect_enum] -> AvaliableTqLimit/32(VPMM_DrivetrainSelect_enum)
  [VTQD_FrAntiBlockAactive_flg] -> OPD Hold/14(VTQD_FrAntiBlockAactive_flg)
  [VTQD_AntiBlockFrActDisTime_s] -> OPD Hold/13(VTQD_AntiBlockFrActDisTime_s)
  [VTQD_RrAntiBlockAactive_flg] -> OPD Hold/12(VTQD_RrAntiBlockAactive_flg)
  [VTQD_AntiBlockRrActDisTime_s] -> OPD Hold/11(VTQD_AntiBlockRrActDisTime_s)
  [VTQD_PreLoadHold_flg] -> AvaliableTqLimit/33(VTQD_PreLoadHold_flg)
  [VTQD_ActBPSPosn_pct] -> AvaliableTqLimit/26(VTQD_ActBPSPosn_pct)
  [VVMC_ActLRSlideRate_pct] -> TqDistribution/18(VVMC_ActLRSlideRate_pct)
  [VVMC_ActRRSlideRate_pct] -> TqDistribution/19(VVMC_ActRRSlideRate_pct)
  VVMC_ActRRSlideRate_pct/1 -> [VVMC_ActRRSlideRate_pct]
  VVMC_ActLRSlideRate_pct/1 -> [VVMC_ActLRSlideRate_pct]
  [VTQD_RegenMode_enum] -> AvaliableTqLimit/34(VTQD_RegenMode_enum)
  [VVMC_ActStESCYaw_degps] -> DriverWhlTqDem/47(VVMC_ActStESCYaw_degps)
  [VINP_YawRate_degps] -> DriverWhlTqDem/46(VINP_YawRate_degps)
  [VINP_SASAngle_Deg] -> DriverWhlTqDem/45(VINP_SASAngle_Deg)
  VVMC_ActStESCYaw_degps/1 -> [VVMC_ActStESCYaw_degps]
  VINP_YawRate_degps/1 -> [VINP_YawRate_degps]
  VINP_SASAngle_Deg/1 -> [VINP_SASAngle_Deg]
  [VTQR_NoABSREDUWhlTqReq_Nm] -> OPD Hold/16(VTQR_NoABSREDUWhlTqReq_Nm)
  [VTQR_NoABSFEDUWhlTqReq_Nm] -> OPD Hold/15(VTQR_NoABSFEDUWhlTqReq_Nm)
  [VINP_FrEDURealTMTq_Nm] -> AvaliableTqLimit/35(VINP_FrEDURealTMTq_Nm)
  [VINP_RrEDURealTMTq_Nm] -> AvaliableTqLimit/36(VINP_RrEDURealTMTq_Nm)
  [VINP_EPBSta_enum] -> OPD Hold/17(VINP_EPBSta_enum)
  OPD Hold/8(VTQD_OPDHoldDelayForP_flg) -> [VTQD_OPDHoldDelayForP_flg]
  [VTQD_OPDHoldDelayForP_flg] -> AvaliableTqLimit/37(VTQD_OPDHoldDelayForP_flg)
  VVMC_CAASActive_flg/1 -> [VVMC_CAASActive_flg]
  [VVMC_CAASActive_flg] -> DriverWhlTqDem/48(VVMC_CAASActive_flg)
  [VTQD_PreLoadPreEn_flg] -> AvaliableTqLimit/38(VTQD_PreLoadPreEn_flg)
  [VVMC_CAASActive_flg] -> AvaliableTqLimit/39(VVMC_CAASActive_flg)
  [VPMM_PwrSta_enum] -> OPD Hold/18(VPMM_PwrSta_enum)
  [VTQD_LowIdleAccPedal_flg] -> OPD Hold/19(VTQD_LowIdleAccPedal_flg)
  [VTQD_ActAPSPosn_pct] -> OPD Hold/20(VTQD_ActAPSPosn_pct)
  VINP_HVBSOH_pct/1 -> [VINP_HVBSOH_pct]
  VINP_HVBCellVoltMax_mV/1 -> [VINP_HVBCellVoltMax_mV]
  VINP_HVBCellVoltMin_mV/1 -> [VINP_HVBCellVoltMin_mV]
  [VINP_HVBSOH_pct] -> AvaliableTqLimit/42(VINP_HVBSOH_pct)
  [VINP_HVBCellVoltMin_mV] -> AvaliableTqLimit/41(VINP_HVBCellVoltMin_mV)
  [VINP_HVBCellVoltMax_mV] -> AvaliableTqLimit/40(VINP_HVBCellVoltMax_mV)
  AvaliableTqLimit/10(VTQD_WhlTqCapGenFr_Nm) -> VTQD_WhlTqCapGenFr_Nm/1
  AvaliableTqLimit/11(VTQD_WhlTqCapGenRr_Nm) -> VTQD_WhlTqCapGenRr_Nm/1
  VINP_HVBattSOC_pct/1 -> [VINP_HVBattSOC_pct]
  [VINP_HVBattSOC_pct] -> Signal for ESC/19(VINP_HVBattSOC_pct)
  OPD Hold/9(VTQD_OPDHoldAllowPark_flg) -> VTQD_OPDHoldAllowPark_flg/1
  [VTQD_FrOPDHoldRelTqGain_Nm] -> OPD Hold/21(VTQD_FrOPDHoldRelTqGain_Nm)
  [VTQD_RrOPDHoldRelTqGain_Nm] -> OPD Hold/22(VTQD_RrOPDHoldRelTqGain_Nm)
  OPD Hold/10(VTQD_OPDHoldLamp_flg) -> VTQD_OPDHoldLamp_flg/1
  VVMC_RearTqRatio_rat/1 -> TqDistribution/20(VVMC_RearTqRatio_rat)
  DriverWhlTqDem/13(VTQD_CreepBaseTqD_Nm) -> VTQD_CreepBaseTqD_Nm/1
  [VVMC_ACCOvrdMemTq_Nm] -> DriverWhlTqDem/49(VVMC_ACCOvrdMemTq_Nm)
  VVMC_ACCOvrdMemTq_Nm/1 -> [VVMC_ACCOvrdMemTq_Nm]
  [VVMC_ADASWhlTqReq_Nm] -> Unit Delay2/1
  Unit Delay2/1 -> DriverWhlTqDem/50(VVMC_LastADASWhlTqReq_Nm)
  [VTQD_OPDHoldActRelTq_Nm] -> DriverWhlTqDem/51(VTQD_OPDHoldActRelTq_Nm)
  OPD Hold/11(VTQD_OPDHoldActRelTq_Nm) -> [VTQD_OPDHoldActRelTq_Nm]
  [VINP_FrPTCSActive_flg] -> OPD Hold/23(VINP_FrPTCSActive_flg)
  [VINP_RrPTCSActive_flg] -> OPD Hold/24(VINP_RrPTCSActive_flg)
  [VINP_ESCActive_flg] -> OPD Hold/25(VINP_ESCActive_flg)
  [VINP_ABSActive_flg] -> OPD Hold/26(VINP_ABSActive_flg)
  VINP_ESCActive_flg/1 -> [VINP_ESCActive_flg]
  VINP_ABSActive_flg/1 -> [VINP_ABSActive_flg]
  [VVMC_APSActive_flg] -> OPD Hold/27(VVMC_APSActive_flg)
  [VINP_IVISnowModeCmd_flg] -> DriverWhlTqDem/52(VINP_IVISnowModeCmd_flg)
  VINP_IVISnowModeCmd_flg/1 -> [VINP_IVISnowModeCmd_flg]
  VINP_VehicleType_enum/1 -> [VINP_VehicleType_enum]
  [VINP_VehicleType_enum] -> AvaliableTqLimit/43(VINP_VehicleType_enum)
  [VDDM_EPBSigErrCFS_flg] -> DriverWhlTqDem/56(VDDM_EPBSigErrCFS_flg)
  [VDDM_EPB1CSErrCFS_flg] -> DriverWhlTqDem/55(VDDM_EPB1CSErrCFS_flg)
  [VDDM_EPB1RCErrCFS_flg] -> DriverWhlTqDem/54(VDDM_EPB1RCErrCFS_flg)
  [VDDM_EPB1NoComCFS_flg] -> DriverWhlTqDem/53(VDDM_EPB1NoComCFS_flg)
  VDDM_EPBSigErrCFS_flg/1 -> [VDDM_EPBSigErrCFS_flg]
  VDDM_EPB1RCErrCFS_flg/1 -> [VDDM_EPB1RCErrCFS_flg]
  VDDM_EPB1CSErrCFS_flg/1 -> [VDDM_EPB1CSErrCFS_flg]
  VDDM_EPB1NoComCFS_flg/1 -> [VDDM_EPB1NoComCFS_flg]
  [VVMC_APSActive_flg] -> ExtTqFuncHandShaking/12(VVMC_APSActive_flg)

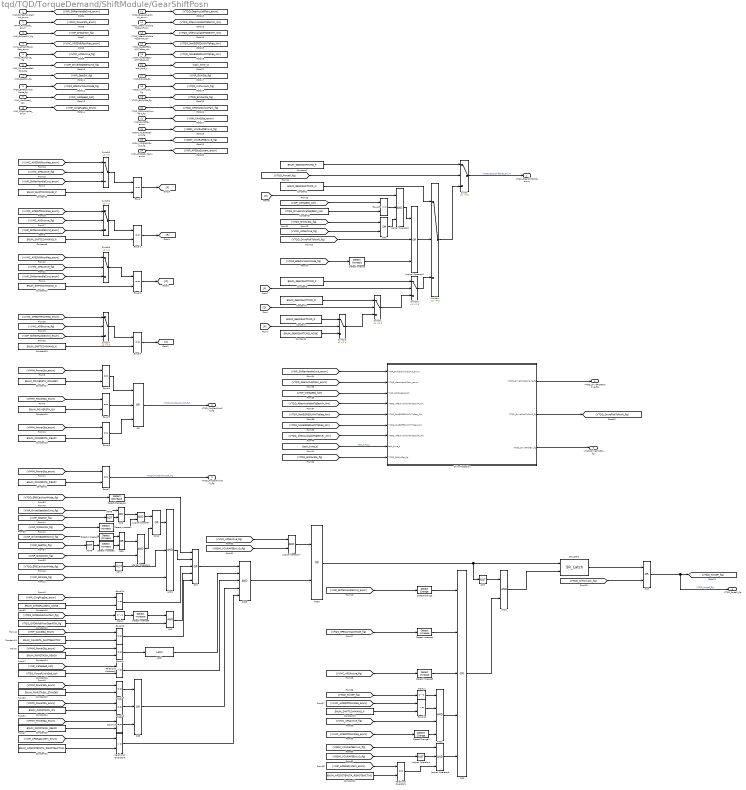
== system tqd/TQD/TorqueDemand/ShiftModule/GearShiftPosn ==
  VINP_ShifterHandleCmd_enum : Inport
  VPMM_PowerSta_enum : Inport  Port=2
  VINP_DrDoorSW_flg : Inport  Port=3
  VVMC_APSShiftPosnReq_enum : Inport  Port=4
  VVMC_APSActive_flg : Inport  Port=5
  VINP_DriverSeatBeltCmd_flg : Inport  Port=6
  VINP_SeatSW_flg : Inport  Port=7
  VTQD_EPBCarWashMode_flg : Inport  Port=8
  VINP_VehSpeed_kph : Inport  Port=9
  VINP_ChrgPlugSta_enum : Inport  Port=10
  VTQD_GearActualPosn_enum : Inport  Port=11
  VTQD_AfterAvailableTqDemFr_Nm : Inport  Port=12
  VTQD_AfterAvailableTqDemRr_Nm : Inport  Port=13
  VTQR_NoABSFEDUWhlTqReq_Nm : Inport  Port=14
  VTQR_NoABSREDUWhlTqReq_Nm : Inport  Port=15
  task_time_s : Inport  Port=16
  VINP_DOASta_flg : Inport  Port=17
  VTQD_IVIPwrLock_flg : Inport  Port=18
  VTQD_BrkSwSta_flg : Inport  Port=19
  VTQD_OPDHoldAllowPark_flg : Inport  Port=20
  VINP_CAASSta_enum : Inport  Port=21
  VDDM_VCURAPSErrLv2_flg : Inport  Port=22
  VDDM_VCURAPSErrLv3_flg : Inport  Port=23
  VINP_APSStaSystem_enum : Inport  Port=24
  AND : Logic  AllPortsSameDT=off  OutDataTypeStr=boolean
  AND1 : Logic  AllPortsSameDT=off  OutDataTypeStr=boolean
  AND2 : Logic  Inputs=4  AllPortsSameDT=off  OutDataTypeStr=boolean
  AND3 : Logic  Operator=OR  AllPortsSameDT=off  OutDataTypeStr=boolean
  AND4 : Logic  Inputs=3  AllPortsSameDT=off  OutDataTypeStr=boolean
  AND5 : Logic  Inputs=5  AllPortsSameDT=off  OutDataTypeStr=boolean
  Constant : Constant  Value=ENUM_GEARSHIFTCMD_R
  Constant1 : Constant  Value=ENUM_POWERSTA_READY
  Constant10 : Constant  Value=KTQD_OPDHoldAllowGearPSW_flg
  Constant11 : Constant  Value=ENUM_CAASSTA_SHIFTGEARTOP
  Constant12 : Constant  Value=ENUM_SHIFTCOMMAND_D
  Constant13 : Constant  Value=ENUM_SHIFTCOMMAND_N
  Constant14 : Constant  Value=ENUM_PWRSTASW_READY
  Constant15 : Constant  Value=ENUM_SHIFTCOMMAND_P
  Constant16 : Constant  Value=ENUM_CHRGPLUGSTA_NONE
  Constant17 : Constant  Value=ENUM_POWERSTA_STANDBY
  Constant18 : Constant  Value=ENUM_POWERSTA_ON
  Constant19 : Constant  Value=ENUM_POWERSTA_READY
  Constant2 : Constant  Value=ENUM_GEARSHIFTCMD_N
  Constant21 : Constant  Value=ENUM_APSSYSTEMSTA_REMOTEACTIVE
  Constant22 : Constant  Value=ENUM_APSSYSTEMSTA_REMOTEACTIVE
  Constant23 : Constant  Value=ENUM_PWRSTASW_STANDBY
  Constant24 : Constant  Value=ENUM_PWRSTASW_ON
  Constant25 : Constant  Value=ENUM_PWRSTASW_READY
  Constant26 : Constant  Value=KTQD_ForcePLimitSpd_kph
  Constant3 : Constant  Value=ENUM_GEARSHIFTCMD_P
  Constant4 : Constant  Value=ENUM_GEARSHIFTCMD_D
  Constant5 : Constant  Value=ENUM_SHIFTCOMMAND_P
  Constant6 : Constant  Value=ENUM_GEARSHIFTCMD_NONE
  Constant7 : Constant  Value=ENUM_GEARSHIFTCMD_P
  Constant8 : Constant  Value=ENUM_SHIFTCOMMAND_R
  Constant9 : Constant  Value=KTQD_DriveProtVehSpdGain_kph
  Delay : Delay  DelayLength=1
  Delay1 : Delay  DelayLength=1
  Detect Change : simulink/Logic and Bit Operations/Detect Change  vinit=0  OutDataTypeStr=boolean
  Detect Change1 : simulink/Logic and Bit Operations/Detect Change  vinit=0  OutDataTypeStr=boolean
  Detect Decrease1 : simulink/Logic and Bit Operations/Detect Decrease  vinit=0.0  OutDataTypeStr=boolean
  Detect Increase{,1..6} (7 alike) : simulink/Logic and Bit Operations/Detect Increase  vinit=0.0  OutDataTypeStr=boolean
  Drive Protection : Subsystem
  Equal{,1..7,9..10,12..13,15} (13 alike) : RelationalOperator  Operator===  OutDataTypeStr=boolean  RndMeth=Simplest
  Equal11 : RelationalOperator  Operator=~=  OutDataTypeStr=boolean  RndMeth=Simplest
  Equal14 : RelationalOperator  Operator=~=  OutDataTypeStr=boolean  RndMeth=Simplest
  Equal8 : RelationalOperator  Operator=<=  OutDataTypeStr=boolean  RndMeth=Simplest
  Latch : hcu_lib/Basic_Blocks/Latch
  Logical Operator : Logic  AllPortsSameDT=off  OutDataTypeStr=boolean
  Logical Operator1 : Logic  AllPortsSameDT=off  OutDataTypeStr=boolean
  Logical Operator2 : Logic  Inputs=3  AllPortsSameDT=off  OutDataTypeStr=boolean
  Logical Operator3 : Logic  Operator=OR  Inputs=3  AllPortsSameDT=off  OutDataTypeStr=boolean
  Logical Operator4 : Logic  Operator=NOT  AllPortsSameDT=off  OutDataTypeStr=boolean
  Logical Operator6 : Logic  Inputs=3  AllPortsSameDT=off  OutDataTypeStr=boolean
  Logical Operator7 : Logic  AllPortsSameDT=off  OutDataTypeStr=boolean
  NOT{,3..5} (4 alike) : Logic  Operator=NOT  AllPortsSameDT=off  OutDataTypeStr=boolean
  OR : Logic  Operator=OR  Inputs=3  AllPortsSameDT=off  OutDataTypeStr=boolean
  OR1 : Logic  Operator=OR  Inputs=5  AllPortsSameDT=off  OutDataTypeStr=boolean
  OR{2..3,6,9..10} (5 alike) : Logic  Operator=OR  AllPortsSameDT=off  OutDataTypeStr=boolean
  OR7 : Logic  Operator=OR  Inputs=5  AllPortsSameDT=off  OutDataTypeStr=boolean
  OR8 : Logic  Operator=OR  Inputs=3  AllPortsSameDT=off  OutDataTypeStr=boolean
  Relational Operator1 : RelationalOperator  Operator===  OutDataTypeStr=boolean  RndMeth=Simplest
  Relational Operator2 : RelationalOperator  Operator=<=  OutDataTypeStr=boolean  RndMeth=Simplest
  Relational Operator3 : RelationalOperator  Operator=~=  OutDataTypeStr=boolean  RndMeth=Simplest
  SR_Latch1 : hcu_lib/Basic_Blocks/SR_Latch
  Switch{,1..4,7} (6 alike) : Switch  Criteria=u2 ~= 0
      Switch1 settings: AttributesFormatString=%<Criteria>
      Switch2 settings: AttributesFormatString=%<Criteria>
      Switch3 settings: AttributesFormatString=%<Criteria>
      Switch4 settings: AttributesFormatString=%<Criteria>
  Switch5 : Switch  Criteria=u2 > Threshold
  Switch6 : Switch  Criteria=u2 > Threshold
  Switch8 : Switch  Criteria=u2 > Threshold
  VTQD_GearShiftCMD_enum : Outport
  VTQD_PwrStaAllowPN_flg : Outport  Port=2
  VTQD_PwrStaAllowDR_flg : Outport  Port=3
  VTQD_DriveProtRemove_flg : Outport  Port=4
  VTQD_DriveProtEn_flg : Outport  Port=5
  VTQD_ForceP_flg : Outport  Port=6
  wires:
  Switch2/1 -> Switch4/3
  Constant2/1 -> Switch4/1
  Switch1/1 -> Switch2/3
  [P] -> Switch2/2
  Constant3/1 -> Switch2/1
  Switch3/1 -> Switch1/3
  Constant/1 -> Switch3/1
  Constant4/1 -> Switch1/1
  [R] -> Switch3/2
  [D] -> Switch1/2
  VINP_ShifterHandleCmd_enum/1 -> [VINP_ShifterHandleCmd_enum]
  Constant5/1 -> Equal/2
  Constant8/1 -> Equal1/2
  Constant12/1 -> Equal2/2
  Constant19/1 -> Equal6/2
  [VPMM_PowerSta_enum] -> Equal6/1
  [VPMM_PowerSta_enum] -> Equal5/1
  [VPMM_PowerSta_enum] -> Equal4/1
  Constant17/1 -> Equal4/2
  Constant18/1 -> Equal5/2
  VPMM_PowerSta_enum/1 -> [VPMM_PowerSta_enum]
  Equal5/1 -> OR/2
  Equal4/1 -> OR/1
  Equal6/1 -> OR/3
  OR/1 -> VTQD_PwrStaAllowPN_flg/1  "VTQD_PwrStaAllowPN_flg"
  [VPMM_PowerSta_enum] -> Equal7/1
  Constant1/1 -> Equal7/2
  Equal7/1 -> VTQD_PwrStaAllowDR_flg/1  "VTQD_PwrStaAllowDR_flg"
  Equal/1 -> [P]
  Equal1/1 -> [R]
  Equal2/1 -> [D]
  Constant6/1 -> Switch3/3
  Switch/1 -> VTQD_GearShiftCMD_enum/1  "VTQD_GearShiftCMD_enum"
  Switch4/1 -> Switch/3
  VINP_DrDoorSW_flg/1 -> [VINP_DrDoorSW_flg]
  [VTQD_ForceP_flg] -> Switch/2
  Constant7/1 -> Switch/1
  VVMC_APSShiftPosnReq_enum/1 -> [VVMC_APSShiftPosnReq_enum]
  VVMC_APSActive_flg/1 -> [VVMC_APSActive_flg]
  Switch5/1 -> Equal/1
  [VVMC_APSActive_flg] -> Switch5/2
  [VVMC_APSShiftPosnReq_enum] -> Switch5/1
  [VVMC_APSShiftPosnReq_enum] -> Switch6/1
  Switch6/1 -> Equal1/1
  [VVMC_APSActive_flg] -> Switch6/2
  [VINP_ShifterHandleCmd_enum] -> Switch6/3
  [VVMC_APSActive_flg] -> Switch7/2
  [VVMC_APSShiftPosnReq_enum] -> Switch8/1
  [VVMC_APSActive_flg] -> Switch8/2
  [VINP_ShifterHandleCmd_enum] -> Switch8/3
  Switch8/1 -> Equal2/1
  VINP_SeatSW_flg/1 -> [VINP_SeatSW_flg]
  VINP_DriverSeatBeltCmd_flg/1 -> [VINP_DriverSeatBeltCmd_flg]
  VTQD_EPBCarWashMode_flg/1 -> [VTQD_EPBCarWashMode_flg]
  VINP_VehSpeed_kph/1 -> [VINP_VehSpeed_kph]
  VINP_ChrgPlugSta_enum/1 -> [VINP_ChrgPlugSta_enum]
  VTQR_NoABSREDUWhlTqReq_Nm/1 -> [VTQR_NoABSREDUWhlTqReq_Nm]
  VTQD_AfterAvailableTqDemFr_Nm/1 -> [VTQD_AfterAvailableTqDemFr_Nm]
  VTQD_GearActualPosn_enum/1 -> [VTQD_GearActualPosn_enum]
  VTQR_NoABSFEDUWhlTqReq_Nm/1 -> [VTQR_NoABSFEDUWhlTqReq_Nm]
  VTQD_AfterAvailableTqDemRr_Nm/1 -> [VTQD_AfterAvailableTqDemRr_Nm]
  task_time_s/1 -> [task_time_s]
  OR6/1 -> Logical Operator/1
  Logical Operator1/1 -> OR10/2
  [VTQD_EPBCarWashMode_flg] -> NOT4/1
  [VPMM_PowerSta_enum] -> Equal15/1
  [VINP_VehSpeed_kph] -> Relational Operator2/1
  Logical Operator/1 -> OR10/1
  Detect Increase3/1 -> OR9/2
  [VINP_DrDoorSW_flg] -> Logical Operator1/2
  [VINP_SeatSW_flg] -> NOT5/1
  [VINP_DrDoorSW_flg] -> Detect Increase1/1
  OR9/1 -> Logical Operator1/1
  Detect Increase2/1 -> OR9/1
  Constant16/1 -> Equal14/2
  NOT5/1 -> Detect Increase3/1
  [VINP_DriverSeatBeltCmd_flg] -> Detect Increase2/1
  Equal12/1 -> OR8/2
  Equal14/1 -> OR7/3
  OR10/1 -> AND4/1
  AND4/1 -> OR7/2
  Equal15/1 -> OR8/1
  Constant23/1 -> Equal15/2
  Constant25/1 -> Equal13/2
  Detect Increase1/1 -> Logical Operator/2
  [VTQD_EPBCarWashMode_flg] -> Detect Decrease1/1
  Constant26/1 -> Relational Operator2/2
  [VPMM_PowerSta_enum] -> Equal13/1
  NOT4/1 -> AND4/2
  Constant24/1 -> Equal12/2
  Equal13/1 -> OR8/3
  [VINP_ChrgPlugSta_enum] -> Equal14/1
  OR7/1 -> AND5/1
  NOT3/1 -> OR6/2
  Detect Decrease1/1 -> OR7/1
  [VINP_DriverSeatBeltCmd_flg] -> OR6/1
  [VINP_SeatSW_flg] -> NOT3/1
  [VPMM_PowerSta_enum] -> Equal12/1
  AND5/1 -> AND3/2
  VINP_DOASta_flg/1 -> [VINP_DOASta_flg]
  [VINP_DOASta_flg] -> AND4/3
  Constant9/1 -> Equal8/2
  [VINP_VehSpeed_kph] -> Equal8/1
  [VTQD_EPBCarWashMode_flg] -> Detect Increase/1
  Detect Increase/1 -> Logical Operator3/3
  Constant13/1 -> Equal9/2
  [VVMC_APSShiftPosnReq_enum] -> Switch7/1
  [VINP_ShifterHandleCmd_enum] -> Switch7/3
  Switch7/1 -> Equal9/1
  Equal9/1 -> [N]
  [N] -> Logical Operator2/1
  Logical Operator2/1 -> Logical Operator3/1
  Logical Operator3/1 -> Switch4/2
  [task_time_s] -> Drive Protection/8(task_time_s)  "task_time_s"
  [VINP_VehSpeed_kph] -> Drive Protection/3(VINP_VehSpeed_kph)
  [VTQD_AfterAvailableTqDemRr_Nm] -> Drive Protection/7(VTQD_AfterAvailableTqDemRr_Nm)
  Drive Protection/1(VTQD_DriveProtRemove_flg) -> VTQD_DriveProtRemove_flg/1
  [VTQD_AfterAvailableTqDemFr_Nm] -> Drive Protection/4(VTQD_AfterAvailableTqDemFr_Nm)
  [VTQR_NoABSREDUWhlTqReq_Nm] -> Drive Protection/5(VTQR_NoABSREDUWhlTqReq_Nm)
  [VTQR_NoABSFEDUWhlTqReq_Nm] -> Drive Protection/6(VTQR_NoABSFEDUWhlTqReq_Nm)
  [VINP_ShifterHandleCmd_enum] -> Drive Protection/1(VINP_ShifterHandleCmd_enum)
  Drive Protection/2(VTQD_DriveProtToPsnN_flg) -> [VTQD_DriveProtToPsnN_flg]
  [VTQD_GearActualPosn_enum] -> Drive Protection/2(VTQD_GearActualPosn_enum)
  VTQD_IVIPwrLock_flg/1 -> [VTQD_IVIPwrLock_flg]
  [VTQD_DriveProtToPsnN_flg] -> Logical Operator3/2
  Drive Protection/3(VTQD_DriveProtEn_flg) -> VTQD_DriveProtEn_flg/1
  [VTQD_IVIPwrLock_flg] -> OR2/2
  SR_Latch1/1 -> OR2/1
  OR2/1 -> VTQD_ForceP_flg/1, [VTQD_ForceP_flg]  "VTQD_ForceP_flg"
  [VPMM_PowerSta_enum] -> Equal3/1
  Equal3/1 -> Latch/1
  Latch/1 -> AND5/2
  Constant14/1 -> Equal3/2
  Relational Operator2/1 -> AND5/3
  OR8/1 -> AND5/4
  [VINP_ShifterHandleCmd_enum] -> Switch5/3
  Equal8/1 -> Logical Operator2/2
  VTQD_BrkSwSta_flg/1 -> [VTQD_BrkSwSta_flg]
  [VTQD_BrkSwSta_flg] -> Drive Protection/9(VTQD_BrkSwSta_flg)
  OR3/1 -> Logical Operator2/3
  [VTQD_BrkSwSta_flg] -> OR3/1
  [VVMC_APSActive_flg] -> OR3/2
  VTQD_OPDHoldAllowPark_flg/1 -> [VTQD_OPDHoldAllowPark_flg]
  AND/1 -> OR7/4
  Detect Increase6/1 -> AND/1
  Constant10/1 -> AND/2
  [VTQD_OPDHoldAllowPark_flg] -> Delay/1
  Delay/1 -> Detect Increase6/1
  VINP_CAASSta_enum/1 -> [VINP_CAASSta_enum]
  [VINP_CAASSta_enum] -> Equal10/1
  Equal10/1 -> OR7/5
  Constant11/1 -> Equal10/2
  [VVMC_APSActive_flg] -> Logical Operator7/1
  [VDDM_VCURAPSErrLv3_flg] -> Logical Operator7/2
  Logical Operator7/1 -> AND3/1
  AND3/1 -> NOT/1, SR_Latch1/1
  [VVMC_APSActive_flg] -> AND2/3
  Delay1/1 -> AND2/1
  [VDDM_VCURAPSErrLv3_flg] -> Logical Operator4/1
  Detect Change/1 -> OR1/1
  Logical Operator4/1 -> Logical Operator6/2
  [VDDM_VCURAPSErrLv2_flg] -> Logical Operator6/1
  [VVMC_APSShiftPosnReq_enum] -> Detect Change1/1
  Detect Increase5/1 -> OR1/3
  Logical Operator6/1 -> OR1/5
  Constant15/1 -> Equal11/2
  [VTQD_ForceP_flg] -> Delay1/1
  [VVMC_APSShiftPosnReq_enum] -> Equal11/1
  Detect Change1/1 -> AND2/4
  NOT/1 -> AND1/1
  OR1/1 -> AND1/2
  AND1/1 -> SR_Latch1/2
  [VTQD_EPBCarWashMode_flg] -> Detect Increase4/1
  Detect Increase4/1 -> OR1/2
  Relational Operator1/1 -> Logical Operator6/3
  Constant21/1 -> Relational Operator1/2
  [VINP_APSStaSystem_enum] -> Relational Operator1/1
  Equal11/1 -> AND2/2
  [VINP_ShifterHandleCmd_enum] -> Detect Change/1
  [VVMC_APSActive_flg] -> Detect Increase5/1
  AND2/1 -> OR1/4
  VDDM_VCURAPSErrLv2_flg/1 -> [VDDM_VCURAPSErrLv2_flg]
  VINP_APSStaSystem_enum/1 -> [VINP_APSStaSystem_enum]
  VDDM_VCURAPSErrLv3_flg/1 -> [VDDM_VCURAPSErrLv3_flg]
  [VINP_APSStaSystem_enum] -> Relational Operator3/1
  Constant22/1 -> Relational Operator3/2
  Relational Operator3/1 -> AND5/5

== system tqd/TQD/TorqueDemand/ShiftModule/P_Button_State_Judge ==
  VINP_ShifterHandleCmd_enum : Inport
  Constant1 : Constant  Value=ENUM_PBUTTON_RELEASED
  Constant12 : Constant  Value=ENUM_SHIFTCOMMAND_D
  Constant15 : Constant  Value=ENUM_SHIFTCOMMAND_N
  Constant2 : Constant  Value=ENUM_PBUTTON_PRESSED
  Constant3 : Constant  Value=ENUM_PBUTTON_INVALID
  Constant4 : Constant  Value=ENUM_SHIFTCOMMAND_NONE
  Constant5 : Constant  Value=ENUM_SHIFTCOMMAND_P
  Constant8 : Constant  Value=ENUM_SHIFTCOMMAND_R
  Equal{,1..4} (5 alike) : RelationalOperator  Operator===  OutDataTypeStr=boolean  RndMeth=Simplest
  Logical Operator : Logic  Operator=OR  Inputs=4  AllPortsSameDT=off  OutDataTypeStr=boolean
  Switch1 : Switch  Criteria=u2 ~= 0
      settings: AttributesFormatString=%<Criteria>
  Switch4 : Switch  Criteria=u2 ~= 0
      settings: AttributesFormatString=%<Criteria>
  VTQD_PButtonSta_enum : Outport
  wires:
  Switch4/1 -> VTQD_PButtonSta_enum/1  "VTQD_PButtonSta_enum"
  VINP_ShifterHandleCmd_enum/1 -> [VINP_ShifterHandleCmd_enum]
  Equal/1 -> [P]
  Constant12/1 -> Equal2/2
  [VINP_ShifterHandleCmd_enum] -> Equal1/1
  Constant8/1 -> Equal1/2
  [VINP_ShifterHandleCmd_enum] -> Equal/1
  Equal2/1 -> Logical Operator/3
  Constant15/1 -> Equal3/2
  Equal3/1 -> Logical Operator/2
  Equal1/1 -> Logical Operator/1
  Constant5/1 -> Equal/2
  [VINP_ShifterHandleCmd_enum] -> Equal3/1
  [VINP_ShifterHandleCmd_enum] -> Equal2/1
  Logical Operator/1 -> [RND]
  [RND] -> Switch4/2
  [P] -> Switch1/2
  Constant1/1 -> Switch4/1
  Switch1/1 -> Switch4/3
  Constant2/1 -> Switch1/1
  Constant3/1 -> Switch1/3
  [VINP_ShifterHandleCmd_enum] -> Equal4/1
  Constant4/1 -> Equal4/2
  Equal4/1 -> Logical Operator/4

== system tqd/TQD/TorqueDemand/ShiftModule/SR_Latch1 ==
  set : Inport
  reset : Inport  Port=2
  Logical Operator : Logic  AllPortsSameDT=off  OutDataTypeStr=boolean
  Logical Operator1 : Logic  Operator=NOT  AllPortsSameDT=off  OutDataTypeStr=boolean
  Switch1 : Switch  Criteria=u2 ~= 0  Threshold=0.5
      settings: AttributesFormatString=<Criteria=%<Criteria>>
  Switch2 : Switch  Criteria=u2 ~= 0  Threshold=0.5
      settings: AttributesFormatString=<Criteria=%<Criteria>>
  Unit Delay : UnitDelay  SampleTime=-1  HasFrameUpgradeWarning=on
  latched : Outport
  wires:
  Switch1/1 -> Unit Delay/1, latched/1
  set/1 -> Switch1/1, Logical Operator/1
  reset/1 -> Switch2/2, Logical Operator1/1
  Unit Delay/1 -> Switch2/3
  Switch2/1 -> Switch1/3
  Logical Operator/1 -> Switch1/2
  Logical Operator1/1 -> Logical Operator/2, Switch2/1
